simulink model "Templates_for_step_and_peel_TestAB_SOCRATES"  (R2025b)
settings: Solver=FixedStepAuto  StartTime=0.0  StopTime=40  FixedStep=Ts  RelTol=1e-3
undefined symbols (not defined in the file or in its folder): CR, LF, motor_IDs, Ts
libraries: simulink_extras x8, dspsigops x8, robotcorelib x5, dspindex x5, dxlSimLibrary x3, dspstat3 x3, instrumentseriallib x3, sldrtlib x1
settings Model: Creator=ziyad  LastModifiedBy=mmm_r
settings SolverCC: EnableFixedStepZeroCrossing=on
settings OptimizationCC: DefaultParameterBehavior=Inlined  EnhancedBackFolding=on  PassReuseOutputArgsThreshold=0.0  MaxStackSize=200000  OptimizeBlockOrder=speed  DifferentSizesBufferReuse=on
settings DebuggingCC: ParameterTunabilityLossMsg=error
settings HardwareCC: ProdBitPerLong=64.0  ProdHWDeviceType=Intel->x86-64 (Linux 64)
settings SFSimCC: MATLABDynamicMemAlloc=off
settings RTWCC: SystemTargetFile=sldrt.tlc  TemplateMakefile=sldrt.tmf  RTWCompilerOptimization=on  Description=Simulink Desktop Real-Time
settings CodeAppCC: ForceParamTrailComments=on  MaxIdLength=95.0  OperatorAnnotations=on
settings SimulinkDesktopRealTimeCC: ExtModeTransport=0.0  ExtModeStaticAllocSize=1000000.0  TargetLibSuffix=_sldrt.a  TargetPreCompLibLocation=C:\Program Files\MATLAB\R2025b\toolbox\sldrt\lib\win64  TargetLangStandard=C89/C90 (ANSI)  MultiwordLength=2048.0  DynamicStringBufferSize=256.0  ParMdlRefBuildCompliant=on  PreserveMATLABNamespacesInGeneratedCode=on  SubcomponentCodeInterfacePackaging=Reusable function

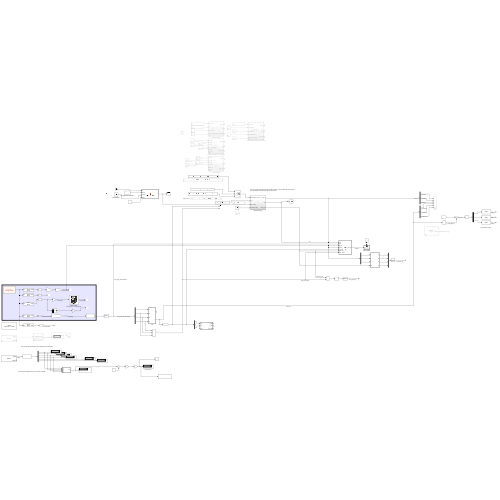
[thumbnail: Simulink's stored preview of the top-level diagram]
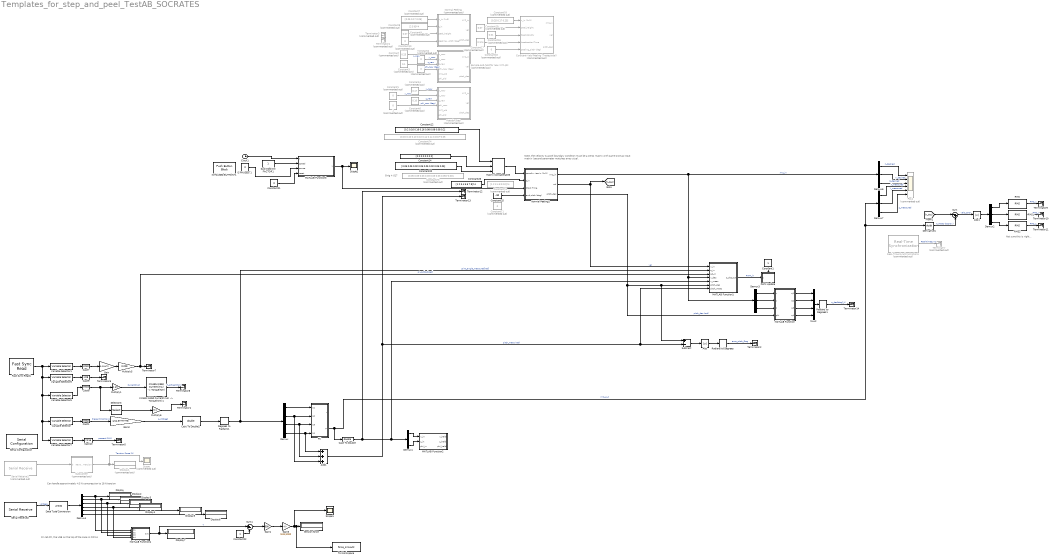
== system Templates_for_step_and_peel_TestAB_SOCRATES ==
  note: Orig +.017
  note: Note, the velocity & accel boundary condition must be a zeros matrix with same size as input matrix (second parameter matches array size).
  note: Not sure this is right...
  note: Can handle approximately 4.5 N compression to 18 N tension
  note: On lab PC, the USB on the top of the case is COM4
  " " : Constant  Commented=on  Value=0
  " 1" : Constant  Commented=on  Value=0
  Abs : Abs  SaturateOnIntegerOverflow=off
  Abs1 : Abs  SaturateOnIntegerOverflow=off
  Add1 : Sum  Inputs=+++
  Cast To Double : DataTypeConversion  OutDataTypeStr=double  SaturateOnIntegerOverflow=off  RndMeth=Floor
  Cast To Double2 : DataTypeConversion  OutDataTypeStr=double  SaturateOnIntegerOverflow=off  RndMeth=Floor
  Cast1 : DataTypeConversion  OutDataTypeStr=int32  SaturateOnIntegerOverflow=off  RndMeth=Floor
  Cast10 : DataTypeConversion  OutDataTypeStr=int16  SaturateOnIntegerOverflow=off  RndMeth=Floor
  Cast7 : DataTypeConversion  OutDataTypeStr=int32  SaturateOnIntegerOverflow=off  RndMeth=Floor
  Cast8 : DataTypeConversion  OutDataTypeStr=int16  SaturateOnIntegerOverflow=off  RndMeth=Floor
  Cast9 : DataTypeConversion  OutDataTypeStr=int8  SaturateOnIntegerOverflow=off  RndMeth=Floor
  Clock1 : Clock
  Constant : Constant  Commented=on  Value=0.25
  Constant-Velo Peeling (Trapezoidal) : Subsystem  Commented=on
  Constant1 : Constant
  Constant{2,5,10..11,16} (5 alike) : Constant  Commented=on  Value=0
  Constant12 : Constant  Value=[0.2 0.16 0.16 0.16 0.08 0.08 0.08 0.2]  VectorParams1D=off
  Constant13 : Constant  Commented=on  Value=[1 2 3 4 8 9 10]*4  VectorParams1D=off
  Constant14 : Constant  Value=[0 0 0 0 0 0 0 0]  VectorParams1D=off
  Constant15 : Constant  Commented=on  Value=0.01
  Constant17 : Constant  Commented=on  Value=0.1*4
  Constant18 : Constant  Commented=on  Value=[0.25 0.17 0.25]  VectorParams1D=off
  Constant19 : Constant  Commented=on  Value=0.07
  Constant20 : Constant  Value=[0.05 0.05 0.02 0.05 0.05 0.02 0.05 0.05]  VectorParams1D=off
  Constant21 : Constant  Value=0
  Constant22 : Constant
  Constant23 : Constant  Commented=on  Value=[0.05 0.05 0.03 0.03 0.03 0.03 0.05]-0.001  VectorParams1D=off
  Constant24 : Constant  Commented=on  Value=[0.15 0.10 0.10 0.10 0.14 0.14 0.15]+0.05  VectorParams1D=off
  Constant25 : Constant  Value=-90
  Constant26 : Constant  Value=[1 2 3 4 5 6 7 8]*4
  Constant3 : Constant  Commented=on  Value=0.1
  Constant4 : Constant  Commented=on  Value=0.17
  Constant6 : Constant  Commented=on  Value=0.10
  Constant7 : Constant  Commented=on  Value=[0.25 0.17 0.25]  VectorParams1D=off
  Constant8 : Constant  Commented=on  Value=[2 5 6]*4  VectorParams1D=off
  Constant9 : Constant  Commented=on  Value=0.07
  Data Type Conversion : DataTypeConversion  OutDataTypeStr=uint32  SaturateOnIntegerOverflow=off  RndMeth=Floor
  Degrees to Radians1 : simulink_extras/Transformations/Degrees to Radians
  Demux : Demux
  Demux{1..3,6..7} (5 alike) : Demux  Outputs=3
  Demux4 : Demux  Outputs=6
  Derivative1 : Derivative
  Display{,2..7} (7 alike) : Display
  Display1 : Display  Commented=on
  FK : MATLAB Function  TreatAsAtomicUnit=on
  Fast Sync Read1 : dxlSimLibrary/Fast Sync Read  lib_name='dxl_x64_c'  group_num_read=group_num_read  ids=motor_IDs  models=motor_models  select_sync_read=select_sync_read  start_address_read_indirect=start_address_read_indirect  Ts=Ts
  Gain : Gain  Gain=0.10472
  Gain1 : Gain  Gain=500
  Gain2 : Gain  Gain=1/11.37777778
  Gain3 : Gain  Gain=9.81/1000
  IS PAUSED BUTTON?1 : PushButtonBlock  ButtonType=Latch  IconOnColor=[0.0, 0.39215686274509803, 0.0]  IconOffColor=[0.0, 1.0, 0.0]  OffValue=0.000000
  IS PAUSED?1 : Constant  Value=0
  MATLAB Function : MATLAB Function  TreatAsAtomicUnit=on
  MATLAB Function1 : MATLAB Function  TreatAsAtomicUnit=on
  MATLAB Function2 : MATLAB Function  TreatAsAtomicUnit=on
  MATLAB Function3 : MATLAB Function  TreatAsAtomicUnit=on
  MATLAB Function4 : MATLAB Function  TreatAsAtomicUnit=on
  Matrix Concatenate3 : Concatenate  NumInputs=3  Mode=Multidimensional array
  Multiply1 : Gain  Gain=2.69  OutDataTypeStr=double
  Multiply5 : Gain  Gain=0.229  OutDataTypeStr=double
  Multiply6 : Gain  Gain=0.1  OutDataTypeStr=double
  Mux2 : Mux
  Normal Peeling : Subsystem  Commented=on
  Normal Peeling1 : Subsystem
  PWM Update : Subsystem  TreatAsAtomicUnit=on
  Pos1 : Scope  Commented=on  NumInputPorts=6
      settings: Title=Time history with a cubic polynomial time law  ActiveDisplayYMinimum=-0.034681761003191973  ActiveDisplayYMaximum=0.29962437658108865  YLabel=Position [m]  DataLoggingVariableName=ScopeData9
  Pseudo-Step : Subsystem  Commented=on
  RMS : dspstat3/RMS  run=off  directionMode=Each column  dimension=1  InputProcessing=Columns as channels (frame based)  reset_popup=None
  RMS1 : dspstat3/RMS  run=off  directionMode=Each column  dimension=1  InputProcessing=Columns as channels (frame based)  reset_popup=None
  RMS2 : dspstat3/RMS  run=off  directionMode=Each column  dimension=1  InputProcessing=Columns as channels (frame based)  reset_popup=None
  Radians to Degrees : simulink_extras/Transformations/Radians to Degrees
  Radians to Degrees1 : simulink_extras/Transformations/Radians to Degrees
  Real-Time Synchronization1 : sldrtlib/Real-Time Synchronization  Commented=on  SampleTime=Ts  MaxMissedTicks=10000  ShowMissedTicks=on  YieldWhenWaiting=off
  SLOWDOWN FACTOR1 : Constant
  Sample-and-hold for new XYZ-phi : Subsystem  Commented=on
  Scope : Scope  Commented=on
      settings: ActiveDisplayYMinimum=-9.866801374604437  ActiveDisplayYMaximum=25.621640031645562
  Scope1 : Scope
      settings: ActiveDisplayYMinimum=-8.896255000609969  ActiveDisplayYMaximum=3.1048120052689088
  Scope2 : Scope
      settings: ActiveDisplayYMinimum=-4.2683249723173073  ActiveDisplayYMaximum=19.036883445445014  DataLoggingVariableName=ScopeData2
  Selector3 : Selector  InputPortWidth=length(motor_IDs)  IndexOptions=Index vector (dialog)  Indices=1  OutputSizes=1
  Serial Configuration : instrumentseriallib/Serial Configuration  Priority=-200000  PortSel=COM3  Port=COM3  ComPort=COM3  BaudRate=115200  DataBits=8  Parity=none  StopBits=1  ByteOrder=little-endian  FlowControl=none  Timeout=10  SimulateUsing=Interpreted execution  BlockInModel=on  aMode=1
  Serial Receive1 : instrumentseriallib/Serial Receive  Priority=1  Commented=on  PortSel=COM3  Port=COM3  ComPort=COM3  DataType=uint8  SaveDataType=uint8  ToggleHeader=off  Header=[255]  ToggleDataSize=on  DataSize=[1 6]  ToggleTerminator=off  Terminator=CR/LF ('\r\n')  CustomTerminator=[]  InputFormat=Column major  EnableBlockingMode=off  ActionDataUnavailable=Output last received value  ActionWhenDataUnavailable=Output last received value  CustomValue=0  SampleTime=Ts  SimulateUsing=Interpreted execution  BlockInModel=on  aMode=1  LibraryInUse=instrumentlib
  Serial Receive2 : instrumentseriallib/Serial Receive  Priority=1  PortSel=COM3  Port=COM3  ComPort=COM3  DataType=uint8  SaveDataType=uint8  ToggleHeader=off  Header=[255]  ToggleDataSize=on  DataSize=[1 6]  ToggleTerminator=off  Terminator=CR/LF ('\r\n')  CustomTerminator=[]  InputFormat=Column major  EnableBlockingMode=off  ActionDataUnavailable=Output last received value  ActionWhenDataUnavailable=Output last received value  CustomValue=0  SampleTime=Ts  SimulateUsing=Interpreted execution  BlockInModel=on  aMode=1  LibraryInUse=instrumentlib
  Subsystem : Subsystem  Commented=on
  Subtract : Sum  Inputs=+-
  Sum : Sum  Inputs=|-+
  Sum1 : Sum  Inputs=|+-
  Terminator : Terminator  Commented=on
  Terminator{1..2,5..14} (12 alike) : Terminator
  Terminator3 : Terminator  Commented=on
  Terminator4 : Terminator  Commented=on
  To Workspace : ToWorkspace  VariableName=force_simout2  SampleTime=-1
  Variable Selector : dspindex/Variable Selector  NumInputs=1  rowsOrCols=Rows  IdxMode=Fixed  Elements=1  ZerOneIdxMode=One-based  errmode=Clip Index  FillMode=on  FillValues=0
  Variable Selector1 : dspindex/Variable Selector  NumInputs=1  rowsOrCols=Rows  IdxMode=Fixed  Elements=2  ZerOneIdxMode=One-based  errmode=Clip Index  FillMode=on  FillValues=0
  Variable Selector5 : dspindex/Variable Selector  NumInputs=1  rowsOrCols=Rows  IdxMode=Fixed  Elements=3  ZerOneIdxMode=One-based  errmode=Clip Index  FillMode=on  FillValues=0
  Variable Selector6 : dspindex/Variable Selector  NumInputs=1  rowsOrCols=Rows  IdxMode=Fixed  Elements=4  ZerOneIdxMode=One-based  errmode=Clip Index  FillMode=on  FillValues=0
  Variable Selector7 : dspindex/Variable Selector  NumInputs=1  rowsOrCols=Rows  IdxMode=Fixed  Elements=5  ZerOneIdxMode=One-based  errmode=Clip Index  FillMode=on  FillValues=0
  "XM430-W350 Current(mA) -> Torque(Nm)1" : dxlSimLibrary/Subsystem/XM430-W350 /XM430-W350 Current(mA) -> Torque(Nm)  SystemSampleTime=-1  VariantActivationTime=update diagram  EmptyChoice=off  PassThrough=off  PassThroughVariantControl=(default)  EmptyChoiceVariantControl=(default)  AllowFlexibleInterface=on  Latency=0  AutoFrameSizeCalculation=off
  tension force : Display
  wires:
  Real-Time Synchronization1/1 -> Terminator/1  "Real-timeSync"
  Constant1/1 -> PWM Update/Enable
  Degrees to Radians1/1 -> MATLAB Function1/2(q_in), Demux/1  "Joint_angle_measured[rad]"
  Demux/2 -> Add1/3, FK/2(q2)
  Demux/1 -> FK/1(q1)
  Demux/4 -> Add1/1, FK/4(q4)
  Demux/3 -> Add1/2, FK/3(q3)
  FK/2(p) -> Derivative1/1, Demux7/1, Cast To Double/1  "XYZ_out"
  Add1/1 -> Terminator13/1, Subtract/2, MATLAB Function1/7(pitch_meas)  "pitch_meas (rad)"
  Demux6/3 -> Pos1/3  "Z_desired"
  Demux6/2 -> Pos1/2  "Y_desired"
  Demux6/1 -> Pos1/1  "X_desired"
  Normal Peeling1/2(vel) -> [V_des], MATLAB Function1/1(v_in)  "vel"
  Normal Peeling1/1(XYZ_in) -> Demux3/1, MATLAB Function1/4(x_des), Demux6/1  "XYZ_in"
  Demux7/3 -> Pos1/6  "Z_measured"
  Demux7/2 -> Pos1/5  "Y_measured"
  Demux7/1 -> Pos1/4  "X_measured"
  "XM430-W350 Current(mA) -> Torque(Nm)1"/1 -> Terminator8/1  "T_pGraph[Nm]"
  Variable Selector5/1 -> Cast8/1
  Multiply6/1 -> Terminator1/1
  Cast9/1 -> Terminator6/1
  Variable Selector1/1 -> Cast7/1
  Selector3/1 -> Multiply6/1
  Cast To Double2/1 -> Degrees to Radians1/1
  Variable Selector/1 -> Cast1/1
  Cast8/1 -> Selector3/1, Multiply1/1
  Cast7/1 -> Gain/1
  Cast1/1 -> Gain2/1  "Present Positions"
  Gain2/1 -> Cast To Double2/1  "q_m[Deg]"
  Multiply5/1 -> MATLAB Function1/3(qd_in), Terminator7/1  "q'_out[rad/sec]"
  Variable Selector6/1 -> Cast9/1
  Multiply1/1 -> "XM430-W350 Current(mA) -> Torque(Nm)1"/1  "Current[mA]"
  Gain/1 -> Multiply5/1
  Normal Peeling1/3(pitch_des) -> MATLAB Function/4(phi), Subtract/1, MATLAB Function1/6(pitch_des)  "pitch_des (rad)"
  MATLAB Function1/1(q_dot_out) -> PWM Update/1(y)  "PWM_in"
  Subtract/1 -> Abs/1
  Abs/1 -> Radians to Degrees/1
  Radians to Degrees/1 -> Terminator2/1  "error_pitch_Deg"
  Variable Selector7/1 -> Cast10/1
  Fast Sync Read1/1 -> Variable Selector5/1, Variable Selector7/1, Variable Selector/1, Variable Selector6/1, Variable Selector1/1
  Cast10/1 -> Terminator5/1  "present PWM"
  Demux1/1 -> MATLAB Function2/1(x_in)
  Demux1/3 -> MATLAB Function2/2(z_in)
  Demux3/1 -> MATLAB Function/1(x)
  Demux3/2 -> MATLAB Function/2(y)
  Demux3/3 -> MATLAB Function/3(z)
  MATLAB Function/1(q1) -> Mux2/1
  MATLAB Function/2(q2) -> Mux2/2
  MATLAB Function/3(q3) -> Mux2/3
  MATLAB Function/4(q4) -> Mux2/4
  Mux2/1 -> Radians to Degrees1/1
  Radians to Degrees1/1 -> Terminator14/1  "q_des[deg]_IK"
  Cast To Double/1 -> Terminator12/1, MATLAB Function1/5(x_meas), Demux1/1
  Subsystem/1(Newton Tension) -> Scope/1, Display1/1  "Tension Force (N)"
  Serial Receive1/1 -> Subsystem/1(b)
  " "/1 -> Sample-and-hold for new XYZ-phi/4(phi_new (deg))  "phi_new (deg)"
  Constant2/1 -> Sample-and-hold for new XYZ-phi/2(y_new)  "y_new"
  Constant3/1 -> Sample-and-hold for new XYZ-phi/3(z_new)  "z_new"
  Constant/1 -> Sample-and-hold for new XYZ-phi/1(x_new)  "x_new"
  Constant5/1 -> Pseudo-Step/2(y_new)  "y_new"
  Constant6/1 -> Pseudo-Step/3(z_new)  "z_new"
  " 1"/1 -> Pseudo-Step/4(phi_new)  "phi_new (deg)"
  Constant4/1 -> Pseudo-Step/1(x_new)  "x_new"
  [V_des] -> Sum/1
  Derivative1/1 -> Sum/2  "V_meas (approx)"
  Demux2/1 -> RMS/1
  Demux2/3 -> RMS2/1
  Demux2/2 -> RMS1/1
  RMS/1 -> Terminator9/1  "RMS_x"
  RMS2/1 -> Terminator11/1  "RMS_z"
  RMS1/1 -> Terminator10/1  "RMS_y"
  Constant10/1 -> Normal Peeling/4(peeling_pitch (deg))
  Constant9/1 -> Normal Peeling/3(peel_height)
  Constant8/1 -> Normal Peeling/2(t_in)
  Constant7/1 -> Normal Peeling/1(x_in (1x3))
  Sum/1 -> Abs1/1  "velo_error"
  Abs1/1 -> Demux2/1
  Constant18/1 -> Constant-Velo Peeling (Trapezoidal)/1(x_in (1x3))
  Constant19/1 -> Constant-Velo Peeling (Trapezoidal)/2(peel_height)
  Constant17/1 -> Constant-Velo Peeling (Trapezoidal)/4(AccelerationTime)
  Constant16/1 -> Constant-Velo Peeling (Trapezoidal)/5(peeling_pitch (deg))
  Constant15/1 -> Constant-Velo Peeling (Trapezoidal)/3(PeakVelocity)
  Matrix Concatenate3/1 -> Normal Peeling1/1(coordinates in (1x3))
  Constant14/1 -> Matrix Concatenate3/2
  SLOWDOWN FACTOR1/1 -> MATLAB Function3/2(speed)
  MATLAB Function3/1(y) -> Scope2/1, Normal Peeling1/3(Clock Time)
  IS PAUSED?1/1 -> MATLAB Function3/3(pause)
  Clock1/1 -> MATLAB Function3/1(t)
  Constant21/1 -> MATLAB Function3/4(reset)
  Sum1/1 -> Gain1/1
  Gain1/1 -> Gain3/1
  Demux4/4 -> MATLAB Function4/4(b4), Display4/1
  Gain3/1 -> Scope1/1, To Workspace/1, tension force/1
  Serial Receive2/1 -> Data Type Conversion/1  "voltage"
  Demux4/1 -> MATLAB Function4/1(b1), Display/1
  Demux4/5 -> Display5/1
  Constant22/1 -> Sum1/2
  Demux4/6 -> Display6/1
  Data Type Conversion/1 -> Demux4/1
  MATLAB Function4/1(out) -> Display7/1, Sum1/1  "V"
  Demux4/3 -> MATLAB Function4/3(b3), Display3/1
  Demux4/2 -> MATLAB Function4/2(b2), Display2/1
  Constant12/1 -> Matrix Concatenate3/1
  Constant20/1 -> Matrix Concatenate3/3
  Constant25/1 -> Normal Peeling1/4(end pitch (deg))
  Constant26/1 -> Normal Peeling1/2(t_in)

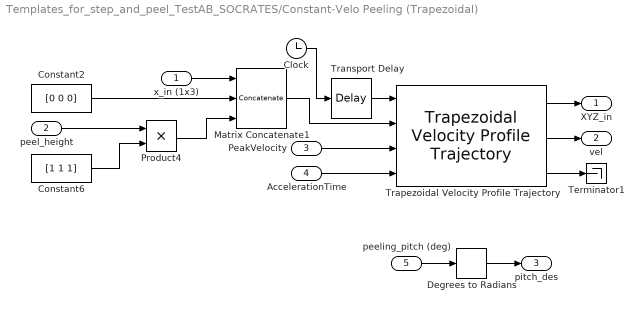
== system Templates_for_step_and_peel_TestAB_SOCRATES/Constant-Velo Peeling (Trapezoidal) ==
  x_in (1x3) : Inport
  peel_height : Inport  Port=2
  PeakVelocity : Inport  Port=3
  AccelerationTime : Inport  Port=4
  peeling_pitch (deg) : Inport  Port=5
  Clock : Clock
  Constant2 : Constant  Value=[0 0 0]  VectorParams1D=off
  Constant6 : Constant  Value=[1 1 1]  VectorParams1D=off
  Degrees to Radians : simulink_extras/Transformations/Degrees to Radians
  Matrix Concatenate1 : Concatenate  NumInputs=3  Mode=Multidimensional array
  Product4 : Product
  Terminator1 : Terminator
  Transport Delay : TransportDelay  DelayTime=2*4
  Trapezoidal Velocity Profile Trajectory : robotcorelib/Trapezoidal Velocity Profile Trajectory  WaypointSource=External  Waypoints=[ 0, -0.5, -1; 0, 0.5, 1 ]  NumParams=2  Parameter1=Peak Velocity  Parameter2=Acceleration Time  ParameterSource=External  PeakVelocity=[ 2; 2 ]  Acceleration=[ 1; 2 ]  EndTime=[ 1; 1 ]  AccelTime=[ 1; 2 ]  SimulateUsing=Interpreted execution
  XYZ_in : Outport
  vel : Outport  Port=2
  pitch_des : Outport  Port=3
  wires:
  peeling_pitch (deg)/1 -> Degrees to Radians/1
  Degrees to Radians/1 -> pitch_des/1
  Trapezoidal Velocity Profile Trajectory/1 -> XYZ_in/1
  Trapezoidal Velocity Profile Trajectory/2 -> vel/1
  Trapezoidal Velocity Profile Trajectory/3 -> Terminator1/1
  AccelerationTime/1 -> Trapezoidal Velocity Profile Trajectory/4
  Matrix Concatenate1/1 -> Trapezoidal Velocity Profile Trajectory/2
  PeakVelocity/1 -> Trapezoidal Velocity Profile Trajectory/3
  x_in (1x3)/1 -> Matrix Concatenate1/1
  Constant2/1 -> Matrix Concatenate1/2
  Product4/1 -> Matrix Concatenate1/3
  Constant6/1 -> Product4/2
  peel_height/1 -> Product4/1
  Clock/1 -> Transport Delay/1
  Transport Delay/1 -> Trapezoidal Velocity Profile Trajectory/1

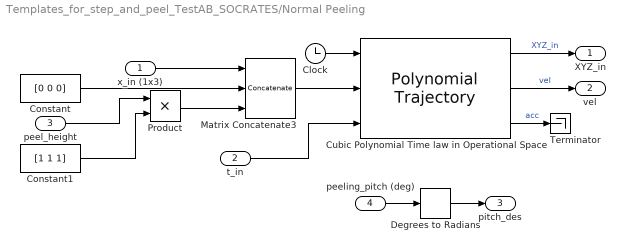
== system Templates_for_step_and_peel_TestAB_SOCRATES/Normal Peeling ==
  x_in (1x3) : Inport
  t_in : Inport  Port=2
  peel_height : Inport  Port=3
  peeling_pitch (deg) : Inport  Port=4
  Clock : Clock
  Constant : Constant  Value=[0 0 0]  VectorParams1D=off
  Constant1 : Constant  Value=[1 1 1]  VectorParams1D=off
  Cubic Polynomial Time law in Operational Space : robotcorelib/Polynomial Trajectory  WaypointSource=External  Waypoints=[0.25,0.25,0.15; 0,0,0; 0.1 ,0.1,0.1]  TimePoints=[1,2,3]  TimeInterval=[ 2, 20 ]  Method=Quintic Polynomial  ParameterSource=Internal  VelocityBoundaryCondition=zeros(3,3)  AccelerationBoundaryCondition=zeros(3,3)  SimulateUsing=Interpreted execution
  Degrees to Radians : simulink_extras/Transformations/Degrees to Radians
  Matrix Concatenate3 : Concatenate  NumInputs=3  Mode=Multidimensional array
  Product : Product
  Terminator : Terminator
  XYZ_in : Outport
  vel : Outport  Port=2
  pitch_des : Outport  Port=3
  wires:
  Clock/1 -> Cubic Polynomial Time law in Operational Space/1
  t_in/1 -> Cubic Polynomial Time law in Operational Space/3
  Product/1 -> Matrix Concatenate3/3
  Constant1/1 -> Product/2
  peel_height/1 -> Product/1
  Constant/1 -> Matrix Concatenate3/2
  x_in (1x3)/1 -> Matrix Concatenate3/1
  Matrix Concatenate3/1 -> Cubic Polynomial Time law in Operational Space/2
  Cubic Polynomial Time law in Operational Space/2 -> vel/1  "vel"
  Cubic Polynomial Time law in Operational Space/3 -> Terminator/1  "acc"
  Cubic Polynomial Time law in Operational Space/1 -> XYZ_in/1  "XYZ_in"
  peeling_pitch (deg)/1 -> Degrees to Radians/1
  Degrees to Radians/1 -> pitch_des/1

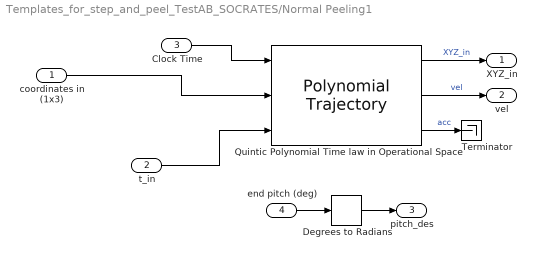
== system Templates_for_step_and_peel_TestAB_SOCRATES/Normal Peeling1 ==
  coordinates in (1x3) : Inport
  t_in : Inport  Port=2
  Clock Time : Inport  Port=3
  end pitch (deg) : Inport  Port=4
  Degrees to Radians : simulink_extras/Transformations/Degrees to Radians
  Quintic Polynomial Time law in Operational Space : robotcorelib/Polynomial Trajectory  WaypointSource=External  Waypoints=[0.25,0.25,0.15; 0,0,0; 0.1 ,0.1,0.1]  TimePoints=[1,2,3]  TimeInterval=[ 2, 20 ]  Method=Quintic Polynomial  ParameterSource=Internal  VelocityBoundaryCondition=zeros(3,8)  AccelerationBoundaryCondition=zeros(3,8)  SimulateUsing=Interpreted execution
  Terminator : Terminator
  XYZ_in : Outport
  vel : Outport  Port=2
  pitch_des : Outport  Port=3
  wires:
  Clock Time/1 -> Quintic Polynomial Time law in Operational Space/1
  t_in/1 -> Quintic Polynomial Time law in Operational Space/3
  coordinates in (1x3)/1 -> Quintic Polynomial Time law in Operational Space/2
  Quintic Polynomial Time law in Operational Space/2 -> vel/1  "vel"
  Quintic Polynomial Time law in Operational Space/3 -> Terminator/1  "acc"
  Quintic Polynomial Time law in Operational Space/1 -> XYZ_in/1  "XYZ_in"
  end pitch (deg)/1 -> Degrees to Radians/1
  Degrees to Radians/1 -> pitch_des/1

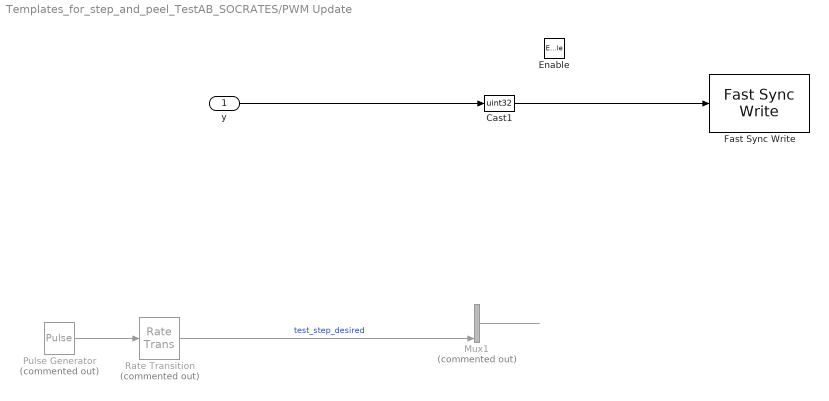
== system Templates_for_step_and_peel_TestAB_SOCRATES/PWM Update ==
  y : Inport
  Enable : EnablePort
  Cast1 : DataTypeConversion  OutMin=0  OutMax=2097150  OutDataTypeStr=uint32  SaturateOnIntegerOverflow=off  RndMeth=Floor
  Fast Sync Write : dxlSimLibrary/Fast Sync Write  Description=|  lib_name=lib_name  group_num_write=group_num_write  ids=motor_IDs  models=motor_models  select_sync_write=select_sync_write  Ts=Ts
      | Dynamixel library for Matlab and Simulink
      | Fast Sync Write function
      | Author: Georgios Andrikopoulos (geoand@kth.se), 2022 
      | Mechatronics & Embedded Control Systems Unit, KTH, Stockholm
  Mux1 : Mux  Commented=on
  Pulse Generator : DiscretePulseGenerator  Commented=on  PulseType=Time based  Amplitude=15  Period=1  PulseWidth=50  PhaseDelay=0.5
  Rate Transition : RateTransition  Commented=on  OutPortSampleTime=Ts
  wires:
  y/1 -> Cast1/1
  Cast1/1 -> Fast Sync Write/1
  Mux1/1 -> ?
  Pulse Generator/1 -> Rate Transition/1
  Rate Transition/1 -> Mux1/4  "test_step_desired"

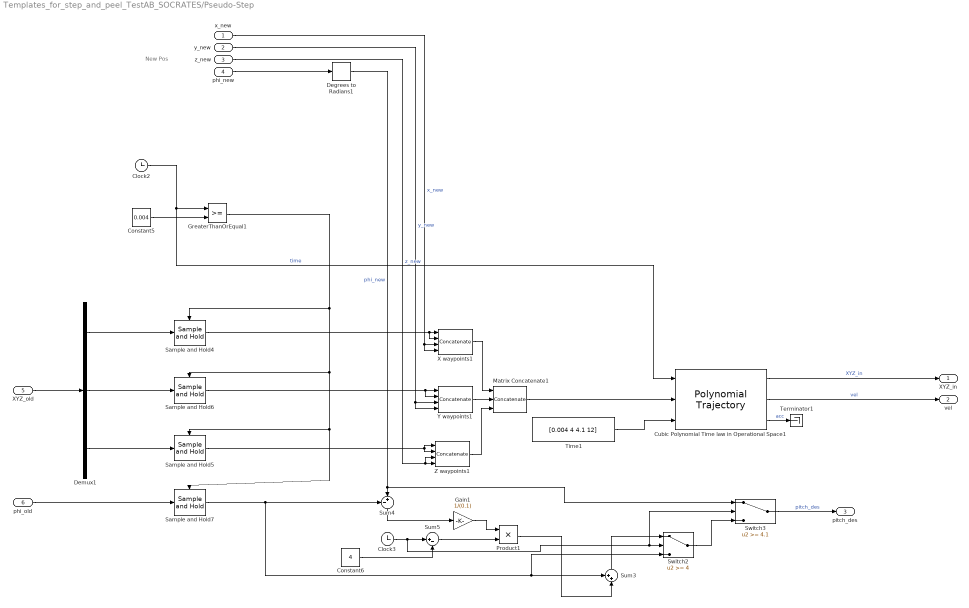
== system Templates_for_step_and_peel_TestAB_SOCRATES/Pseudo-Step ==
  note: New Pos
  x_new : Inport
  y_new : Inport  Port=2
  z_new : Inport  Port=3
  phi_new : Inport  Port=4
  XYZ_old : Inport  Port=5
  phi_old : Inport  Port=6
  Clock2 : Clock
  Clock3 : Clock
  Constant5 : Constant  Value=0.004
  Constant6 : Constant  Value=4
  Cubic Polynomial Time law in Operational Space1 : robotcorelib/Polynomial Trajectory  WaypointSource=External  Waypoints=[0.25,0.25,0.15; 0,0,0; 0.1 ,0.1,0.1]  TimePoints=[1,2,3]  TimeInterval=[ 2, 20 ]  Method=Quintic Polynomial  ParameterSource=Internal  VelocityBoundaryCondition=zeros(3,4)  AccelerationBoundaryCondition=zeros( 3,4)  SimulateUsing=Interpreted execution
  Degrees to Radians1 : simulink_extras/Transformations/Degrees to Radians
  Demux1 : Demux  Outputs=3
  Gain1 : Gain  Gain=1/(0.1)
  GreaterThanOrEqual1 : RelationalOperator  OutDataTypeStr=boolean  RndMeth=Simplest  InputSameDT=off
  Matrix Concatenate1 : Concatenate  NumInputs=3  Mode=Multidimensional array
  Product1 : Product
  Sample and Hold4 : dspsigops/Sample and Hold  trig=Rising edge  initCond=0.233  latchinput=off
  Sample and Hold5 : dspsigops/Sample and Hold  trig=Rising edge  initCond=0.026  latchinput=off
  Sample and Hold6 : dspsigops/Sample and Hold  trig=Rising edge  initCond=0  latchinput=off
  Sample and Hold7 : dspsigops/Sample and Hold  trig=Rising edge  initCond=0  latchinput=off
  Sum3 : Sum  Inputs=++|
  Sum4 : Sum  Inputs=-+|
  Sum5 : Sum  Inputs=|+-
  Switch2 : Switch  Threshold=4  SaturateOnIntegerOverflow=off  InputSameDT=off
  Switch3 : Switch  Threshold=4.1  SaturateOnIntegerOverflow=off  InputSameDT=off
  Terminator1 : Terminator
  Time1 : Constant  Value=[0.004 4 4.1 12]
  X waypoints1 : Concatenate  NumInputs=4  Mode=Multidimensional array  ConcatenateDimension=2
  Y waypoints1 : Concatenate  NumInputs=4  Mode=Multidimensional array  ConcatenateDimension=2
  Z waypoints1 : Concatenate  NumInputs=4  Mode=Multidimensional array  ConcatenateDimension=2
  XYZ_in : Outport
  vel : Outport  Port=2
  pitch_des : Outport  Port=3
  wires:
  XYZ_old/1 -> Demux1/1
  Time1/1 -> Cubic Polynomial Time law in Operational Space1/3
  Z waypoints1/1 -> Matrix Concatenate1/3
  Cubic Polynomial Time law in Operational Space1/3 -> Terminator1/1  "acc"
  Cubic Polynomial Time law in Operational Space1/2 -> vel/1  "vel"
  Cubic Polynomial Time law in Operational Space1/1 -> XYZ_in/1  "XYZ_in"
  Matrix Concatenate1/1 -> Cubic Polynomial Time law in Operational Space1/2
  X waypoints1/1 -> Matrix Concatenate1/1
  Sample and Hold5/1 -> Z waypoints1/1, Z waypoints1/2
  Gain1/1 -> Product1/1
  Demux1/3 -> Sample and Hold5/1
  Sum3/1 -> Switch2/1
  Constant5/1 -> GreaterThanOrEqual1/2
  Demux1/2 -> Sample and Hold6/1
  Constant6/1 -> Sum5/2
  Sample and Hold7/1 -> Switch2/3, Sum3/1, Sum4/1
  GreaterThanOrEqual1/1 -> Sample and Hold7/Trigger, Sample and Hold5/Trigger, Sample and Hold6/Trigger, Sample and Hold4/Trigger
  Switch3/1 -> pitch_des/1  "pitch_des"
  phi_new/1 -> Degrees to Radians1/1
  Clock3/1 -> Sum5/1, Switch3/2, Switch2/2
  phi_old/1 -> Sample and Hold7/1
  Sample and Hold6/1 -> Y waypoints1/2, Y waypoints1/1
  Degrees to Radians1/1 -> Switch3/1, Sum4/2  "phi_new"
  Clock2/1 -> Cubic Polynomial Time law in Operational Space1/1, GreaterThanOrEqual1/1  "time"
  Y waypoints1/1 -> Matrix Concatenate1/2
  Sum4/1 -> Gain1/1
  Sum5/1 -> Product1/2
  Product1/1 -> Sum3/2
  Sample and Hold4/1 -> X waypoints1/2, X waypoints1/1
  y_new/1 -> Y waypoints1/4, Y waypoints1/3  "y_new"
  z_new/1 -> Z waypoints1/3, Z waypoints1/4  "z_new"
  Switch2/1 -> Switch3/3
  x_new/1 -> X waypoints1/3, X waypoints1/4  "x_new"
  Demux1/1 -> Sample and Hold4/1

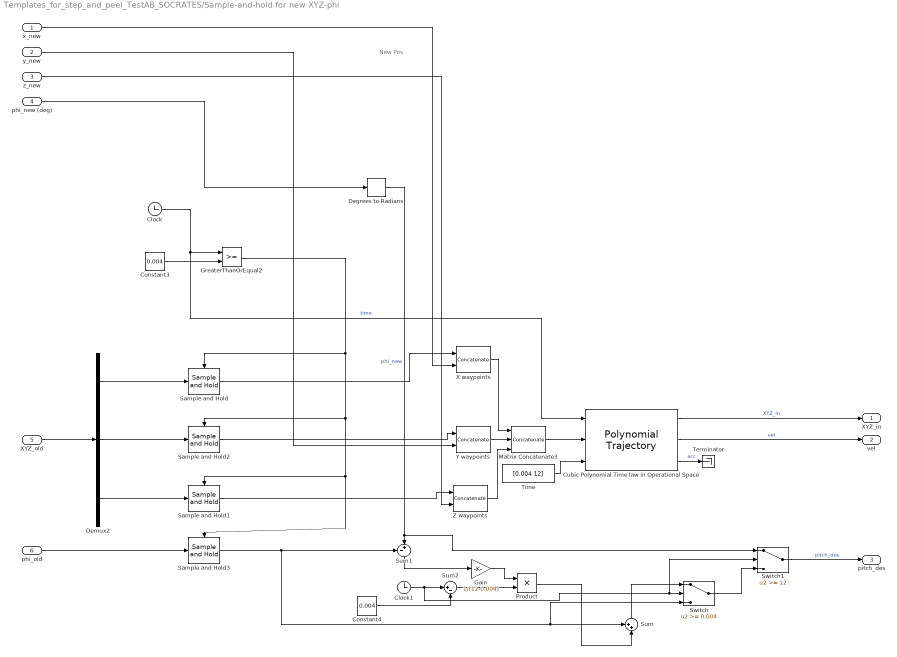
== system Templates_for_step_and_peel_TestAB_SOCRATES/Sample-and-hold for new XYZ-phi ==
  note: New Pos
  x_new : Inport
  y_new : Inport  Port=2
  z_new : Inport  Port=3
  phi_new (deg) : Inport  Port=4
  XYZ_old : Inport  Port=5
  phi_old : Inport  Port=6
  Clock : Clock
  Clock1 : Clock
  Constant3 : Constant  Value=0.004
  Constant4 : Constant  Value=0.004
  Cubic Polynomial Time law in Operational Space : robotcorelib/Polynomial Trajectory  WaypointSource=External  Waypoints=[0.25,0.25,0.15; 0,0,0; 0.1 ,0.1,0.1]  TimePoints=[1,2,3]  TimeInterval=[ 2, 20 ]  Method=Quintic Polynomial  ParameterSource=Internal  VelocityBoundaryCondition=zeros(3,2)  AccelerationBoundaryCondition=zeros( 3,2 )  SimulateUsing=Interpreted execution
  Degrees to Radians : simulink_extras/Transformations/Degrees to Radians
  Demux2 : Demux  Outputs=3
  Gain : Gain  Gain=1/(12-0.004)
  GreaterThanOrEqual2 : RelationalOperator  OutDataTypeStr=boolean  RndMeth=Simplest  InputSameDT=off
  Matrix Concatenate3 : Concatenate  NumInputs=3  Mode=Multidimensional array
  Product : Product
  Sample and Hold : dspsigops/Sample and Hold  trig=Rising edge  initCond=0.233  latchinput=off
  Sample and Hold1 : dspsigops/Sample and Hold  trig=Rising edge  initCond=0.026  latchinput=off
  Sample and Hold2 : dspsigops/Sample and Hold  trig=Rising edge  initCond=0  latchinput=off
  Sample and Hold3 : dspsigops/Sample and Hold  trig=Rising edge  initCond=0  latchinput=off
  Sum : Sum  Inputs=++|
  Sum1 : Sum  Inputs=-+|
  Sum2 : Sum  Inputs=|+-
  Switch : Switch  Threshold=0.004  SaturateOnIntegerOverflow=off  InputSameDT=off
  Switch1 : Switch  Threshold=12  SaturateOnIntegerOverflow=off  InputSameDT=off
  Terminator : Terminator
  Time : Constant  Value=[0.004 12]
  X waypoints : Concatenate  Mode=Multidimensional array  ConcatenateDimension=2
  Y waypoints : Concatenate  Mode=Multidimensional array  ConcatenateDimension=2
  Z waypoints : Concatenate  Mode=Multidimensional array  ConcatenateDimension=2
  XYZ_in : Outport
  vel : Outport  Port=2
  pitch_des : Outport  Port=3
  wires:
  Switch1/1 -> pitch_des/1  "pitch_des"
  Clock/1 -> Cubic Polynomial Time law in Operational Space/1, GreaterThanOrEqual2/1  "time"
  X waypoints/1 -> Matrix Concatenate3/1
  Switch/1 -> Switch1/3
  y_new/1 -> Y waypoints/2
  Demux2/3 -> Sample and Hold1/1
  GreaterThanOrEqual2/1 -> Sample and Hold3/Trigger, Sample and Hold1/Trigger, Sample and Hold2/Trigger, Sample and Hold/Trigger
  Sample and Hold3/1 -> Switch/3, Sum/1, Sum1/1
  Time/1 -> Cubic Polynomial Time law in Operational Space/3
  x_new/1 -> X waypoints/2
  Degrees to Radians/1 -> Switch1/1, Sum1/2  "phi_new"
  Clock1/1 -> Sum2/1, Switch1/2, Switch/2
  Sample and Hold/1 -> X waypoints/1
  XYZ_old/1 -> Demux2/1
  Sum1/1 -> Gain/1
  Cubic Polynomial Time law in Operational Space/1 -> XYZ_in/1  "XYZ_in"
  Gain/1 -> Product/1
  Cubic Polynomial Time law in Operational Space/3 -> Terminator/1  "acc"
  Demux2/2 -> Sample and Hold2/1
  z_new/1 -> Z waypoints/2
  Y waypoints/1 -> Matrix Concatenate3/2
  Sample and Hold2/1 -> Y waypoints/1
  Cubic Polynomial Time law in Operational Space/2 -> vel/1  "vel"
  Matrix Concatenate3/1 -> Cubic Polynomial Time law in Operational Space/2
  Constant3/1 -> GreaterThanOrEqual2/2
  Constant4/1 -> Sum2/2
  Sum/1 -> Switch/1
  Z waypoints/1 -> Matrix Concatenate3/3
  Demux2/1 -> Sample and Hold/1
  Sum2/1 -> Product/2
  Sample and Hold1/1 -> Z waypoints/1
  Product/1 -> Sum/2
  phi_new (deg)/1 -> Degrees to Radians/1
  phi_old/1 -> Sample and Hold3/1

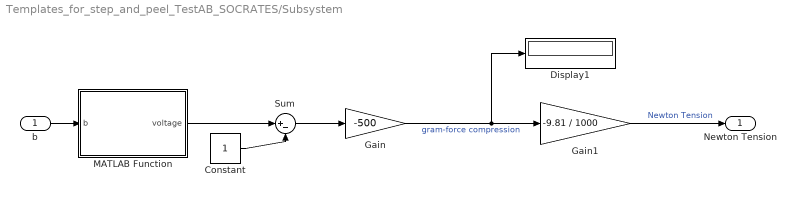
== system Templates_for_step_and_peel_TestAB_SOCRATES/Subsystem ==
  b : Inport
  Constant : Constant
  Display1 : Display
  Gain : Gain  Gain=-500
  Gain1 : Gain  Gain=-9.81 / 1000
  MATLAB Function : MATLAB Function  TreatAsAtomicUnit=on
  Sum : Sum  Inputs=|+-
  Newton Tension : Outport
  wires:
  Gain/1 -> Display1/1, Gain1/1  "gram-force compression"
  b/1 -> MATLAB Function/1(b)
  Sum/1 -> Gain/1
  MATLAB Function/1(voltage) -> Sum/1
  Gain1/1 -> Newton Tension/1  "Newton Tension"
  Constant/1 -> Sum/2

== matlab function Templates_for_step_and_peel_TestAB_SOCRATES/MATLAB Function ==
  data: x input; q1 output; y input; z input; phi input; q2 output; q3 output; q4 output
function [q1,q2,q3,q4] = fcn(x,y,z,phi)
    % Link parameters
    a2 = 0.13; a3 = 0.124; a4 = 0.0815;
    d1 = 0.077;

    % Base angle
    q1 = atan2(y,x);

    % Wrist center position sqrt(x^2 + z^2)
    pwx = sqrt(x^2 + y^2) - a4*cos(phi);
    pwz = z - d1 - a4*sin(phi);

    % Distance from shoulder to wrist center
    dist = sqrt(pwx^2 + pwz^2);

    %Reachability check
    if dist > (a2 + a3) || dist < abs(a2 - a3)
        error('Target point is outside the reachable workspace');
    end

    % Compute q3
    c3 = (pwx^2 + pwz^2 - a2^2 - a3^2)/(2*a2*a3);
    s3 = -sqrt(1 - c3^2); % (-)elbow-up (use +s3 for elbow-down)
    q3 = atan2(s3,c3);
% beta = atan2(a3*s3, a2 + a3*c3)
% gamma = atan2(pwz,pwx)
    % Compute q2
    q2 = atan2(pwz,pwx) - atan2(a3*s3, a2 + a3*c3);
    % Compute q4
    q4 = phi - (q2 + q3);
   
end

== matlab function Templates_for_step_and_peel_TestAB_SOCRATES/MATLAB Function1 ==
  data: v_in input; q_dot_out output; q_in input; qd_in input; x_des input; x_meas input; pitch_des input; pitch_meas input
function q_dot_out = fcn(v_in, q_in, qd_in, x_des, x_meas, pitch_des, pitch_meas)
v_in       = double(v_in);
q_in       = double(q_in);
qd_in      = double(qd_in(:));
x_des      = double(x_des);
x_meas     = double(x_meas);
pitch_des  = double(pitch_des);
pitch_meas = double(pitch_meas);

Ts = 1/500;
l1 = 0.130;
l2 = 0.124;
l3 = 0.0815;

q_dot_lim = 600.0;

persistent int_x_err int_pitch_err
if isempty(int_x_err)
    int_x_err     = zeros(3,1);
    int_pitch_err = 0;
end

q1 = q_in(1);
q2 = q_in(2);
q3 = q_in(3);
q4 = q_in(4);

s1   = sin(q1);   c1   = cos(q1);
s2   = sin(q2);   c2   = cos(q2);
s23  = sin(q2+q3); c23  = cos(q2+q3);
s234 = sin(q2+q3+q4); c234 = cos(q2+q3+q4);

R = l1*c2 + l2*c23 + l3*c234;
J = zeros(3,4);
J(:,1) = [-s1*R; c1*R; 0];
J(:,2) = [-c1*(l1*s2 + l2*s23 + l3*s234);
          -s1*(l1*s2 + l2*s23 + l3*s234);
           l1*c2 + l2*c23 + l3*c234];
J(:,3) = [-c1*(l2*s23 + l3*s234);
          -s1*(l2*s23 + l3*s234);
           l2*c23 + l3*c234];
J(:,4) = [-c1*l3*s234; -s1*l3*s234; l3*c234];

J_o = [0 1 1 1];
J_aug = [J; J_o];

JJt = J_aug * J_aug';
mu  = sqrt(max(det(JJt), 0));
mu_thresh   = 0.01;
lambda_min  = 1e-3;
lambda_max  = 5e-2;
if mu < mu_thresh
    lambda = lambda_max * (1 - (mu/mu_thresh)^2);
else
    lambda = lambda_min;
end
J_pinv = J_aug' / (JJt + lambda^2*eye(4));

x_err     = x_des     - x_meas;
pitch_err = pitch_des - pitch_meas;

v_meas    = J_aug * qd_in;
v_err_lin = v_in - v_meas(1:3);
omega_err = -v_meas(4);

% Kp_x     = diag([1800, 1700, 2500]);
% Kd_x     = diag([  20,   20,   30]);
% Ki_x     = diag([ 285,  285,  300]);

Kp_x     = diag([4.3250,    4.3250,    9.7311]*10^3); %diag([50, 50, 50]*1.5*1.5*1.5*1.5*1.5*1.5*1.5*1.5*1.5*1.5);
Kd_x     = diag([  0,   0,   0]);
Ki_x     = diag([ 20,  20,  20]);

Kp_pitch =  3.4172*10^3*1.5;%200*1.5*1.5*1.5*1.5*1.5*1.5*1.5;
Kd_pitch = 0;
Ki_pitch = 10;

v_lin_cmd = v_in ...
            + Kp_x  * x_err ...
            + Kd_x  * v_err_lin ...
            + Ki_x  * int_x_err;
omega_cmd =   Kp_pitch * pitch_err ...
            + Kd_pitch * omega_err ...
            + Ki_pitch * int_pitch_err;

z_bias = 22;
v_lin_cmd(3) = v_lin_cmd(3) + z_bias;

v_cmd = [v_lin_cmd; omega_cmd];

q_dot_unsat = J_pinv * v_cmd;
q_dot_out = max(min(q_dot_unsat, q_dot_lim), -q_dot_lim);

%q_dot_out = q_dot_unsat;

int_x_err     = int_x_err     + x_err     * Ts;
int_pitch_err = int_pitch_err + pitch_err * Ts;

int_x_err     = max(min(int_x_err,     0.02), -0.02);
int_pitch_err = max(min(int_pitch_err, 0.2 ), -0.2 );

end

== matlab function Templates_for_step_and_peel_TestAB_SOCRATES/Subsystem/MATLAB Function ==
  data: b input; voltage output
function voltage = fcn(b)
    raw = uint32(b(1)) + uint32(b(2))*256 + uint32(b(3))*65536 + uint32(b(4))*16777216;
    voltage = double(typecast(raw, 'single'));
end

== matlab function Templates_for_step_and_peel_TestAB_SOCRATES/FK ==
  data: q1 input; r output; q2 input; q3 input; q4 input; p output
function [r,p] = fcn(q1,q2,q3,q4)

% D-H parameters. 
a1 = 0;     alpha1 = 1/2;  d1 = 0.077;
a2 = 0.13;  alpha2 = 0;     d2 = 0;
a3 = 0.124; alpha3 = 0;     d3 = 0;
a4 = 0.0815; alpha4 = 0;     d4 = 0;

T = @(theta, d, a, alpha) [cos(theta), -sin(theta)*cospi(alpha),  sin(theta)*sinpi(alpha), a*cos(theta);
                           sin(theta),  cos(theta)*cospi(alpha), -cos(theta)*sinpi(alpha), a*sin(theta);
                           0,           sinpi(alpha),             cospi(alpha),            d;
                           0,           0,                      0,                     1];

T1 = T(q1, d1, a1, alpha1);
T2 = T(q2, d2, a2, alpha2);
T3 = T(q3, d3, a3, alpha3);
T4 = T(q4, d4, a4, alpha4);


T = T1*T2*T3*T4;
r = T(1:3,1:3);
p = T(1:3,4);

== matlab function Templates_for_step_and_peel_TestAB_SOCRATES/MATLAB Function2 ==
  data: x_in input; x_held output; z_in input; phi_in input; z_held output; phi_held output
function [x_held, z_held, phi_held] = fcn(x_in, z_in, phi_in)
%#codegen
persistent x0 z0 phi0 captured
if isempty(captured)
    x0       = x_in;
    z0       = z_in;
    phi0     = phi_in;
    captured = true;
end
x_held   = x0;
z_held   = z0;
phi_held = phi0;
end

== matlab function Templates_for_step_and_peel_TestAB_SOCRATES/MATLAB Function3 ==
  data: t input; y output; speed input; pause input; reset input
function y = advanced_clock(t, speed, pause, reset)

persistent last_t scaled_time initialized

if isempty(initialized) || reset
    last_t = t;
    scaled_time = 0;
    initialized = true;
end

dt = t - last_t;

if speed <= 0
    speed = 1;
end

if ~pause
    scaled_time = scaled_time + dt * speed;
end

y = scaled_time;

last_t = t;

== matlab function Templates_for_step_and_peel_TestAB_SOCRATES/MATLAB Function4 ==
  data: b1 input; out output; b2 input; b3 input; b4 input
function out = fcn(b1, b2, b3, b4)
    raw = uint32(b1) + uint32(b2)*256 + uint32(b3)*256^2 + uint32(b4)*256^3;
    out = double(typecast(raw, 'single'));
end
